simulink model "Eg5_3"  (R2018a)
settings: Solver=VariableStepAuto  StartTime=0.0  StopTime=10.0  RelTol=1e-3
settings Model: Creator=wangluo  LastModifiedBy=wangluo

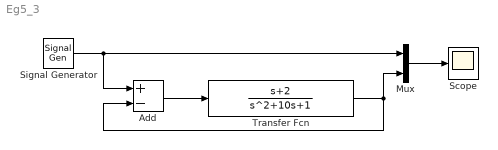
== system Eg5_3 ==
  Add : Sum  Inputs=+-
  Mux : Mux  Inputs=2
  Scope : Scope
  Signal Generator : SignalGenerator  WaveForm=sawtooth  Frequency=1/4
  Transfer Fcn : TransferFcn  Numerator=[1 2]  Denominator=[1 10 1]
  wires:
  Add/1 -> Transfer Fcn/1
  Signal Generator/1 -> Add/1, Mux/1
  Transfer Fcn/1 -> Add/2, Mux/2
  Mux/1 -> Scope/1
